simulink model "probarLinealidad"  (R2018a)
settings: Solver=VariableStepAuto  StartTime=0.0  StopTime=25  RelTol=1e-3
values from neighbouring files (symbols this model uses):
  C = 2267    [paramsLinealizado.m]
  H_l = 1.05    [paramsLinealizado.m]
  n0_S = 1322    [paramsLinealizado.m]
  P_cp = 1924    [paramsLinealizado.m]
libraries: simulink x9
settings Model: Creator=wenap  LastModifiedBy=chris
settings DataIOCC: ReturnWorkspaceOutputs=on
settings SFSimCC: SimUseLocalCustomCode=on
settings RTWCC: RTWUseLocalCustomCode=on

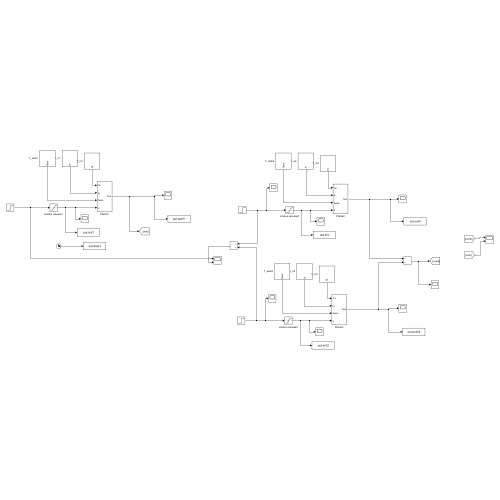
[thumbnail: Simulink's stored preview of the top-level diagram]
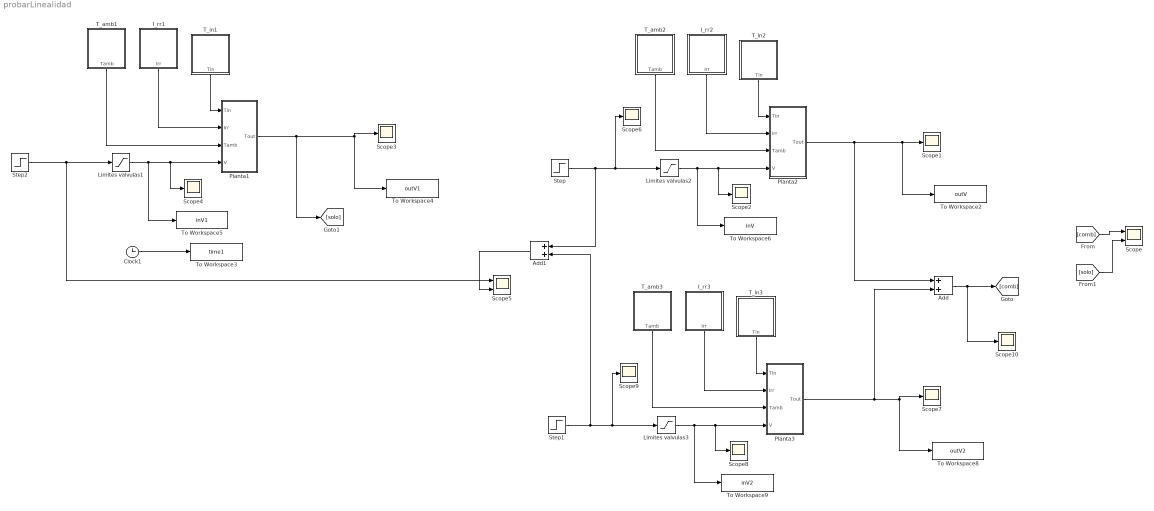
== system probarLinealidad ==
  Add : Sum
  Add1 : Sum
  Clock1 : Clock
  I_rr1 : Subsystem
  I_rr2 : Subsystem
  I_rr3 : Subsystem
  Limites valvulas1 : Saturate  UpperLimit=12  LowerLimit=2
  Limites valvulas2 : Saturate  UpperLimit=12  LowerLimit=2
  Limites valvulas3 : Saturate  UpperLimit=12  LowerLimit=2
  Planta1 : Subsystem
  Planta2 : Subsystem
  Planta3 : Subsystem
  Scope : Scope  NumInputPorts=2
  Scope{1..4,6..10} (9 alike) : Scope
  Scope5 : Scope  NumInputPorts=2
  Step : Step  Time=5  Before=2  After=5  SampleTime=0
  Step1 : Step  Time=5  Before=2  After=7  SampleTime=0
  Step2 : Step  Time=5  Before=4  After=12  SampleTime=0
  T_amb1 : Subsystem
  T_amb2 : Subsystem
  T_amb3 : Subsystem
  T_in1 : Subsystem
  T_in2 : Subsystem
  T_in3 : Subsystem
  To Workspace2 : ToWorkspace  VariableName=outV  SaveFormat=Timeseries  SampleTime=-1
  To Workspace3 : ToWorkspace  VariableName=time1  SampleTime=-1
  To Workspace4 : ToWorkspace  VariableName=outV1  SaveFormat=Timeseries  SampleTime=-1
  To Workspace5 : ToWorkspace  VariableName=inV1  SaveFormat=Timeseries  SampleTime=-1
  To Workspace6 : ToWorkspace  VariableName=inV  SaveFormat=Timeseries  SampleTime=-1
  To Workspace8 : ToWorkspace  VariableName=outV2  SaveFormat=Timeseries  SampleTime=-1
  To Workspace9 : ToWorkspace  VariableName=inV2  SaveFormat=Timeseries  SampleTime=-1
  wires:
  I_rr1/1(Irr) -> Planta1/2(Irr)
  Planta1/1(Tout) -> [solo], Scope3/1, To Workspace4/1
  Clock1/1 -> To Workspace3/1
  Limites valvulas1/1 -> To Workspace5/1, Scope4/1, Planta1/4(V)
  T_in1/1(Tin) -> Planta1/1(Tin)
  T_amb1/1(Tamb) -> Planta1/3(Tamb)
  Step2/1 -> Scope5/1, Limites valvulas1/1
  Step/1 -> Add1/1, Scope6/1, Limites valvulas2/1
  Planta2/1(Tout) -> Add/1, Scope1/1, To Workspace2/1
  T_amb2/1(Tamb) -> Planta2/3(Tamb)
  T_in2/1(Tin) -> Planta2/1(Tin)
  Limites valvulas2/1 -> To Workspace6/1, Scope2/1, Planta2/4(V)
  I_rr2/1(Irr) -> Planta2/2(Irr)
  Step1/1 -> Add1/2, Scope9/1, Limites valvulas3/1
  Limites valvulas3/1 -> To Workspace9/1, Scope8/1, Planta3/4(V)
  T_amb3/1(Tamb) -> Planta3/3(Tamb)
  Planta3/1(Tout) -> Add/2, Scope7/1, To Workspace8/1
  I_rr3/1(Irr) -> Planta3/2(Irr)
  T_in3/1(Tin) -> Planta3/1(Tin)
  Add1/1 -> Scope5/2
  Add/1 -> Scope10/1, [comb]
  [comb] -> Scope/1
  [solo] -> Scope/2

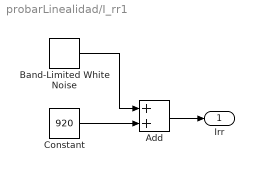
== system probarLinealidad/I_rr1 ==
  Add : Sum
  Band-Limited White Noise : simulink/Sources/Band-Limited White Noise  Cov=[0.0001]  Ts=1  seed=[2]
  Constant : Constant  Value=920
  Irr : Outport
  wires:
  Constant/1 -> Add/2
  Add/1 -> Irr/1
  Band-Limited White Noise/1 -> Add/1

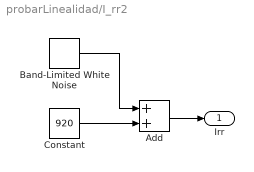
== system probarLinealidad/I_rr2 ==
  Add : Sum
  Band-Limited White Noise : simulink/Sources/Band-Limited White Noise  Cov=[0.0001]  Ts=1  seed=[2]
  Constant : Constant  Value=920
  Irr : Outport
  wires:
  Constant/1 -> Add/2
  Add/1 -> Irr/1
  Band-Limited White Noise/1 -> Add/1

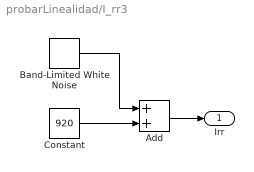
== system probarLinealidad/I_rr3 ==
  Add : Sum
  Band-Limited White Noise : simulink/Sources/Band-Limited White Noise  Cov=[0.0001]  Ts=1  seed=[2]
  Constant : Constant  Value=920
  Irr : Outport
  wires:
  Constant/1 -> Add/2
  Add/1 -> Irr/1
  Band-Limited White Noise/1 -> Add/1

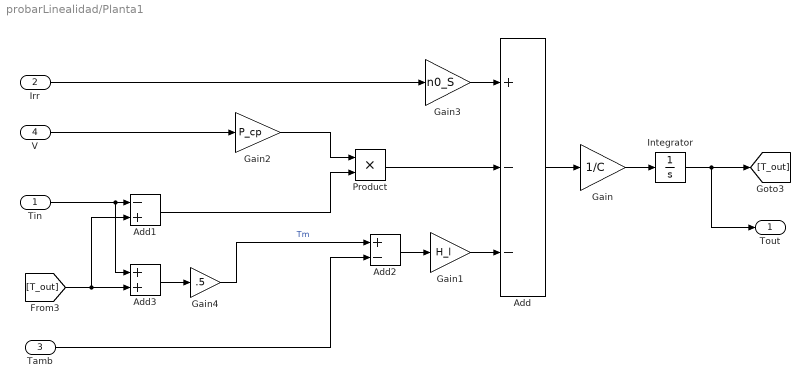
== system probarLinealidad/Planta1 ==
  Tin : Inport
  Irr : Inport  Port=2
  Tamb : Inport  Port=3
  V : Inport  Port=4
  Add : Sum  Inputs=+--
  Add1 : Sum  Inputs=-+
  Add2 : Sum  Inputs=+-
  Add3 : Sum
  Gain : Gain  Gain=1/C
  Gain1 : Gain  Gain=H_l
  Gain2 : Gain  Gain=P_cp
  Gain3 : Gain  Gain=n0_S
  Gain4 : Gain  Gain=.5
  Integrator : Integrator
  Product : Product
  Tout : Outport
  wires:
  Gain2/1 -> Product/1
  Gain3/1 -> Add/1
  Add2/1 -> Gain1/1
  Add1/1 -> Product/2
  Gain/1 -> Integrator/1
  Integrator/1 -> Tout/1, [T_out]
  Add3/1 -> Gain4/1
  Tamb/1 -> Add2/2
  [T_out] -> Add3/2, Add1/2
  Tin/1 -> Add3/1, Add1/1
  Add/1 -> Gain/1
  Product/1 -> Add/2
  Gain1/1 -> Add/3
  Irr/1 -> Gain3/1
  Gain4/1 -> Add2/1  "Tm"
  V/1 -> Gain2/1

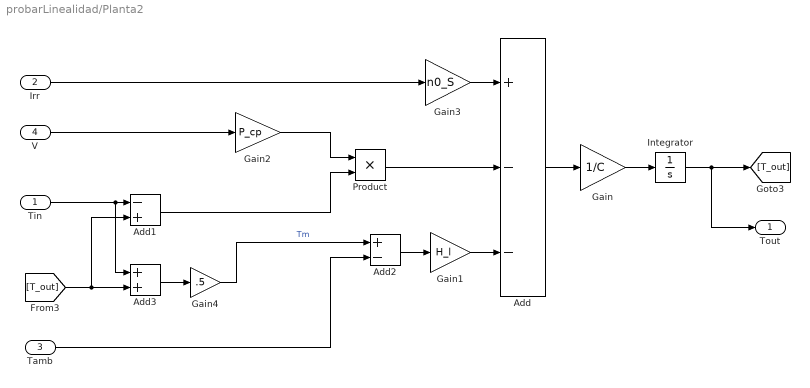
== system probarLinealidad/Planta2 ==
  Tin : Inport
  Irr : Inport  Port=2
  Tamb : Inport  Port=3
  V : Inport  Port=4
  Add : Sum  Inputs=+--
  Add1 : Sum  Inputs=-+
  Add2 : Sum  Inputs=+-
  Add3 : Sum
  Gain : Gain  Gain=1/C
  Gain1 : Gain  Gain=H_l
  Gain2 : Gain  Gain=P_cp
  Gain3 : Gain  Gain=n0_S
  Gain4 : Gain  Gain=.5
  Integrator : Integrator
  Product : Product
  Tout : Outport
  wires:
  Gain2/1 -> Product/1
  Gain3/1 -> Add/1
  Add2/1 -> Gain1/1
  Add1/1 -> Product/2
  Gain/1 -> Integrator/1
  Integrator/1 -> Tout/1, [T_out]
  Add3/1 -> Gain4/1
  Tamb/1 -> Add2/2
  [T_out] -> Add3/2, Add1/2
  Tin/1 -> Add3/1, Add1/1
  Add/1 -> Gain/1
  Product/1 -> Add/2
  Gain1/1 -> Add/3
  Irr/1 -> Gain3/1
  Gain4/1 -> Add2/1  "Tm"
  V/1 -> Gain2/1

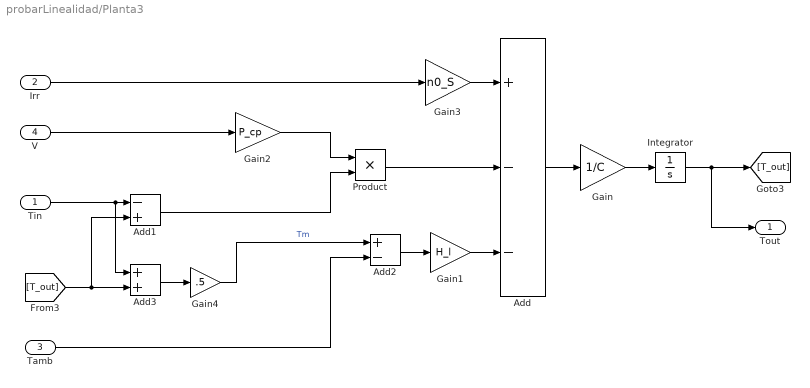
== system probarLinealidad/Planta3 ==
  Tin : Inport
  Irr : Inport  Port=2
  Tamb : Inport  Port=3
  V : Inport  Port=4
  Add : Sum  Inputs=+--
  Add1 : Sum  Inputs=-+
  Add2 : Sum  Inputs=+-
  Add3 : Sum
  Gain : Gain  Gain=1/C
  Gain1 : Gain  Gain=H_l
  Gain2 : Gain  Gain=P_cp
  Gain3 : Gain  Gain=n0_S
  Gain4 : Gain  Gain=.5
  Integrator : Integrator
  Product : Product
  Tout : Outport
  wires:
  Gain2/1 -> Product/1
  Gain3/1 -> Add/1
  Add2/1 -> Gain1/1
  Add1/1 -> Product/2
  Gain/1 -> Integrator/1
  Integrator/1 -> Tout/1, [T_out]
  Add3/1 -> Gain4/1
  Tamb/1 -> Add2/2
  [T_out] -> Add3/2, Add1/2
  Tin/1 -> Add3/1, Add1/1
  Add/1 -> Gain/1
  Product/1 -> Add/2
  Gain1/1 -> Add/3
  Irr/1 -> Gain3/1
  Gain4/1 -> Add2/1  "Tm"
  V/1 -> Gain2/1

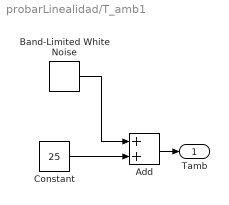
== system probarLinealidad/T_amb1 ==
  Add : Sum
  Band-Limited White Noise : simulink/Sources/Band-Limited White Noise  Cov=[0.0001]  Ts=0.1  seed=[1]
  Constant : Constant  Value=25
  Tamb : Outport
  wires:
  Constant/1 -> Add/2
  Add/1 -> Tamb/1
  Band-Limited White Noise/1 -> Add/1

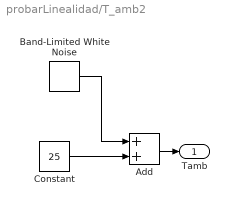
== system probarLinealidad/T_amb2 ==
  Add : Sum
  Band-Limited White Noise : simulink/Sources/Band-Limited White Noise  Cov=[0.0001]  Ts=0.1  seed=[1]
  Constant : Constant  Value=25
  Tamb : Outport
  wires:
  Constant/1 -> Add/2
  Add/1 -> Tamb/1
  Band-Limited White Noise/1 -> Add/1

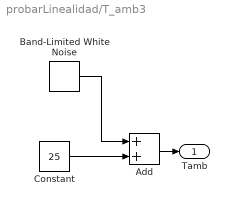
== system probarLinealidad/T_amb3 ==
  Add : Sum
  Band-Limited White Noise : simulink/Sources/Band-Limited White Noise  Cov=[0.0001]  Ts=0.1  seed=[1]
  Constant : Constant  Value=25
  Tamb : Outport
  wires:
  Constant/1 -> Add/2
  Add/1 -> Tamb/1
  Band-Limited White Noise/1 -> Add/1

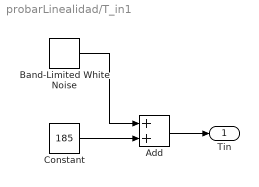
== system probarLinealidad/T_in1 ==
  Add : Sum
  Band-Limited White Noise : simulink/Sources/Band-Limited White Noise  Cov=[0.0001]  Ts=1  seed=[3]
  Constant : Constant  Value=185
  Tin : Outport
  wires:
  Add/1 -> Tin/1
  Constant/1 -> Add/2
  Band-Limited White Noise/1 -> Add/1

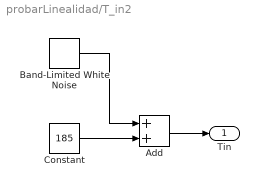
== system probarLinealidad/T_in2 ==
  Add : Sum
  Band-Limited White Noise : simulink/Sources/Band-Limited White Noise  Cov=[0.0001]  Ts=1  seed=[3]
  Constant : Constant  Value=185
  Tin : Outport
  wires:
  Add/1 -> Tin/1
  Constant/1 -> Add/2
  Band-Limited White Noise/1 -> Add/1

== system probarLinealidad/T_in3 ==
  Add : Sum
  Band-Limited White Noise : simulink/Sources/Band-Limited White Noise  Cov=[0.0001]  Ts=1  seed=[3]
  Constant : Constant  Value=185
  Tin : Outport
  wires:
  Add/1 -> Tin/1
  Constant/1 -> Add/2
  Band-Limited White Noise/1 -> Add/1
